simulink model "ClosedLoop_CqCsc"  (R2024a)
settings: Solver=VariableStepAuto  StartTime=0.0  StopTime=10.0  RelTol=1e-3
libraries: RCTblocks x4
settings Model: Creator=Thoma  LastModifiedBy=Thoma

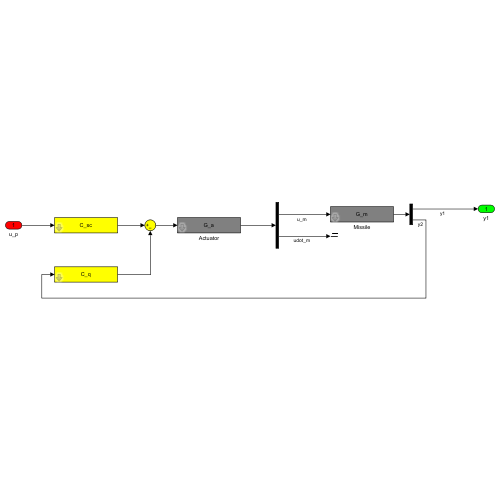
[thumbnail: Simulink's stored preview of the top-level diagram]
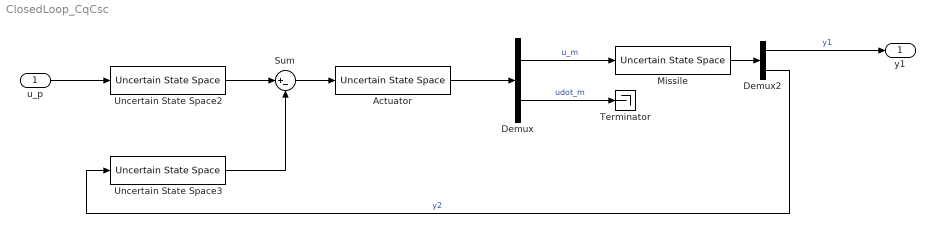
== system ClosedLoop_CqCsc ==
  u_p : Inport
  Actuator : RCTblocks/Uncertain State Space  Tag=USS  USystem=G_a  UValue=[]  X0=[]  uX0=[]
  Demux : Demux  Outputs=2
  Demux2 : Demux  Outputs=2
  Missile : RCTblocks/Uncertain State Space  Tag=USS  USystem=G_m  UValue=[]  X0=[]  uX0=[]
  Sum : Sum  Inputs=|+-
  Terminator : Terminator
  Uncertain State Space2 : RCTblocks/Uncertain State Space  Tag=USS  USystem=C_sc  UValue=[]  X0=[]  uX0=[]
  Uncertain State Space3 : RCTblocks/Uncertain State Space  Tag=USS  USystem=C_q  UValue=[]  X0=[]  uX0=[]
  y1 : Outport
  wires:
  Demux/1 -> Missile/1  "u_m"
  Missile/1 -> Demux2/1
  Demux2/1 -> y1/1  "y1"
  u_p/1 -> Uncertain State Space2/1
  Demux2/2 -> Uncertain State Space3/1  "y2"
  Actuator/1 -> Demux/1
  Sum/1 -> Actuator/1
  Uncertain State Space3/1 -> Sum/2
  Uncertain State Space2/1 -> Sum/1
  Demux/2 -> Terminator/1  "udot_m"
